simulink model "TQ2m"  (Simulink 8.0)
settings: Solver=FixedStepDiscrete  StartTime=0.0  StopTime=inf  FixedStep=0.0025  RelTol=1e-3
undefined symbols (not defined in the file): Serial_Port, Standard_Devices
libraries: simulink x2, rtwinlib x2
Description:
  | Vectorized Quantizer C-MEX S-function
settings Model: Creator=The MathWorks Inc.  LastModifiedBy=x  SimulationMode=external  ExtModeTrigDuration=10000
settings SolverCC: PositivePriorityOrder=on
settings DataIOCC: LimitDataPoints=off  SignalLoggingSaveFormat=ModelDataLogs
settings OptimizationCC: BlockReduction=off  BooleanDataType=off  InitFltsAndDblsToZero=on
settings DebuggingCC: SaveWithParameterizedLinksMsg=none  SignalResolutionControl=TryResolveAllWithWarning  SolverPrmCheckMsg=none  MultiTaskDSMMsg=warning  MultiTaskCondExecSysMsg=none  FcnCallInpInsideContextMsg=UseLocalSettings
settings HardwareCC: ProdIntDivRoundTo=Zero  ProdEndianess=LittleEndian  ProdHWDeviceType=Generic->32-bit x86 compatible  TargetIntDivRoundTo=Zero  TargetEndianess=LittleEndian  TargetHWDeviceType=MATLAB Host  ProdEqTarget=off
settings SFSimCC: SimCustomHeaderCode=|
  | advapi32.dll
  | comctl32.dll
  | comdlg32.dll
  | gdi32.dll
  | kernel32.dll
  | netapi32.dll
  | shell32.dll
  | shlwapi.dll
  | user32.dll
  | WindowsCodecs.dll
settings SFSimCC: SimUserLibraries=|
  | NtDsAPI.Lib
  | NTMSAPI.Lib
  | NtQuery.Lib
  | windowscodecs.lib
settings RTWCC: SystemTargetFile=rtwin.tlc  TemplateMakefile=rtwin.tmf  Description=Real-Time Windows Target  ProcessScript=rtwin_make_rtw_hook  IncludeERTFirstTime=on  RTWCompilerOptimization=On
settings RTWCC: CustomLibrary=|
  | kernel32.lib
  | kernel32.dll
settings CodeAppCC: MaxIdLength=95  CustomSymbolStrType=$N$R$M_T  InternalIdentifier=Shortened
settings RTWinTargetCC: TargetLibSuffix=_rtwin.lib  TargetPreCompLibLocation=C:\Program Files\MATLAB\R2012b\toolbox\rtw\targets\rtwin\lib\win64  CodeReplacementLibrary=ANSI_C  RTWinDir=C:/PROGRA~1/MATLAB/R2012b/toolbox/rtw/targets/rtwin  TargetArch=win64

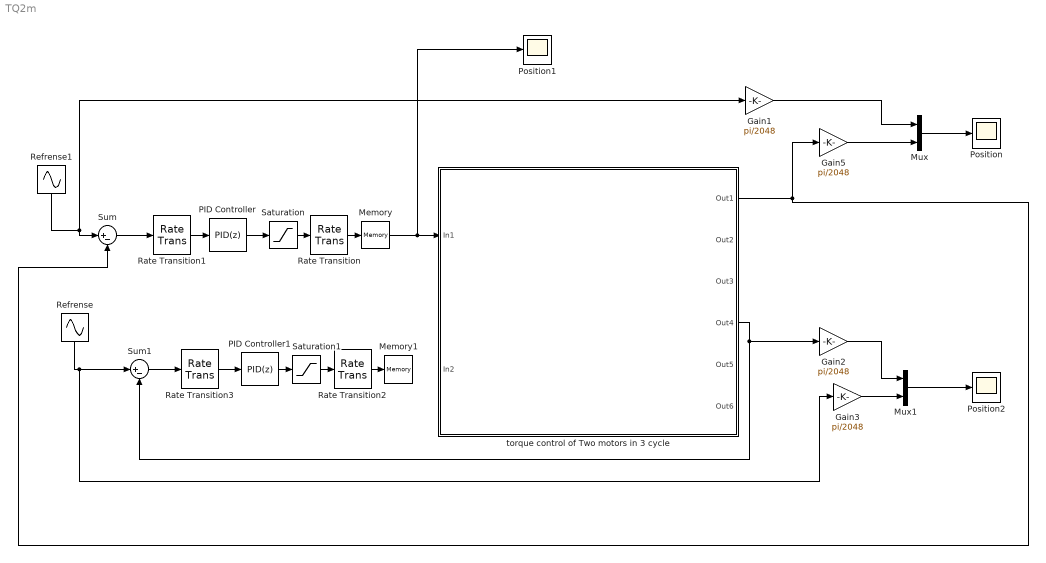
== system TQ2m ==
  Gain{1..3,5} (4 alike) : Gain  Gain=pi/2048
  Memory : Memory
  Memory1 : Memory
  Mux : Mux  Inputs=2
  Mux1 : Mux  Inputs=2
  PID Controller : simulink/Continuous/PID Controller  Controller=PID  TimeDomain=Discrete-time  SampleTime=0.01  IntegratorMethod=Forward Euler  FilterMethod=Forward Euler  Form=Parallel  P=0.002  I=0.01  D=0.00005  N=100  InitialConditionSource=internal  InitialConditionForIntegrator=0  InitialConditionForFilter=0  ExternalReset=none  LimitOutput=off  UpperSaturationLimit=inf  LowerSaturationLimit=-inf  LinearizeAsGain=on  AntiWindupMode=none  Kb=1  TrackingMode=off  Kt=1  PParamMin=[]  PParamMax=[]  IParamMin=[]  IParamMax=[]  DParamMin=[]  DParamMax=[]  NParamMin=[]  NParamMax=[]  KbParamMin=[]  KbParamMax=[]  KtParamMin=[]  KtParamMax=[]  POutMin=[]  POutMax=[]  IOutMin=[]  IOutMax=[]  DOutMin=[]  DOutMax=[]  NOutMin=[]  NOutMax=[]  KbOutMin=[]  KbOutMax=[]  KtOutMin=[]  KtOutMax=[]  IntegratorOutMin=[]  IntegratorOutMax=[]  FilterOutMin=[]  FilterOutMax=[]  SumOutMin=[]  SumOutMax=[]  SumI1OutMin=[]  SumI1OutMax=[]  SumI2OutMin=[]  SumI2OutMax=[]  SumI3OutMin=[]  SumI3OutMax=[]  SumDOutMin=[]  SumDOutMax=[]  SaturationOutMin=[]  SaturationOutMax=[]  IntegratorContinuousStateAttributes=''  IntegratorStateMustResolveToSignalObject=off  IntegratorRTWStateStorageClass=Auto  FilterContinuousStateAttributes=''  FilterStateMustResolveToSignalObject=off  FilterRTWStateStorageClass=Auto
      link override Filter: IntegratorMethod=Integration: Forward Euler  gainval=1.0  ExternalReset=none  InitialConditionSource=internal  InitialCondition=InitialConditionForFilter  InitialConditionMode=State only (most efficient)  SampleTime=-1  OutMin=FilterOutMin  OutMax=FilterOutMax  OutDataTypeStr=FilterOutDataTypeStr  LimitOutput=off  UpperSaturationLimit=inf  LowerSaturationLimit=-inf  ShowSaturationPort=off  ShowStatePort=off
      link override Filter: StateMustResolveToSignalObject=off  RTWStateStorageClass=Auto
  PID Controller1 : simulink/Continuous/PID Controller  Controller=PID  TimeDomain=Discrete-time  SampleTime=0.01  IntegratorMethod=Forward Euler  FilterMethod=Forward Euler  Form=Parallel  P=0.002  I=0.01  D=0.00005  N=100  InitialConditionSource=internal  InitialConditionForIntegrator=0  InitialConditionForFilter=0  ExternalReset=none  LimitOutput=off  UpperSaturationLimit=inf  LowerSaturationLimit=-inf  LinearizeAsGain=on  AntiWindupMode=none  Kb=1  TrackingMode=off  Kt=1  PParamMin=[]  PParamMax=[]  IParamMin=[]  IParamMax=[]  DParamMin=[]  DParamMax=[]  NParamMin=[]  NParamMax=[]  KbParamMin=[]  KbParamMax=[]  KtParamMin=[]  KtParamMax=[]  POutMin=[]  POutMax=[]  IOutMin=[]  IOutMax=[]  DOutMin=[]  DOutMax=[]  NOutMin=[]  NOutMax=[]  KbOutMin=[]  KbOutMax=[]  KtOutMin=[]  KtOutMax=[]  IntegratorOutMin=[]  IntegratorOutMax=[]  FilterOutMin=[]  FilterOutMax=[]  SumOutMin=[]  SumOutMax=[]  SumI1OutMin=[]  SumI1OutMax=[]  SumI2OutMin=[]  SumI2OutMax=[]  SumI3OutMin=[]  SumI3OutMax=[]  SumDOutMin=[]  SumDOutMax=[]  SaturationOutMin=[]  SaturationOutMax=[]  IntegratorContinuousStateAttributes=''  IntegratorStateMustResolveToSignalObject=off  IntegratorRTWStateStorageClass=Auto  FilterContinuousStateAttributes=''  FilterStateMustResolveToSignalObject=off  FilterRTWStateStorageClass=Auto
      link override Filter: IntegratorMethod=Integration: Forward Euler  gainval=1.0  ExternalReset=none  InitialConditionSource=internal  InitialCondition=InitialConditionForFilter  InitialConditionMode=State only (most efficient)  SampleTime=-1  OutMin=FilterOutMin  OutMax=FilterOutMax  OutDataTypeStr=FilterOutDataTypeStr  LimitOutput=off  UpperSaturationLimit=inf  LowerSaturationLimit=-inf  ShowSaturationPort=off  ShowStatePort=off
      link override Filter: StateMustResolveToSignalObject=off  RTWStateStorageClass=Auto
  Position : Scope
      settings: TimeRange=10  YMin=2.2  YMax=3.9  SaveName=ScopeData5
  Position1 : Scope
      settings: TimeRange=10  YMin=-0.3  YMax=0.25
  Position2 : Scope
      settings: TimeRange=10  YMin=2.3  YMax=3.9  SaveName=ScopeData9
  Rate Transition : RateTransition
  Rate Transition1 : RateTransition  OutPortSampleTime=0.01
  Rate Transition2 : RateTransition
  Rate Transition3 : RateTransition  OutPortSampleTime=0.01
  Refrense : Sin  Amplitude=500  Bias=2000  Frequency=1.5
  Refrense1 : Sin  Amplitude=500  Bias=2000  Frequency=1.5
  Saturation : Saturate  UpperLimit=6  LowerLimit=-6
  Saturation1 : Saturate  UpperLimit=6  LowerLimit=-6
  Sum : Sum  Inputs=|+-
  Sum1 : Sum  Inputs=|+-
  torque control of Two motors in 3 cycle : Subsystem  TreatAsAtomicUnit=on  mask(MX64R Real Time Windows Target){p1=3, p2=1}
      mask prompts: p1 "Dynamixel ID 1"; p2 "Dynamixel ID 2"
      mask help:
      | This Block is desined for torque control of two Dynamixel motor (MX64R )in real time workshop
      | please be advised with the following issue:
      | Caution1>> change Status Return Level to 1 in EEprom inorder to receive status packet just for read command.
      | Caution2>> It is recommended that Return Delay Time be set as the minimum value within the allowed range of Main Controller.
      | Caution3>> Total sample time for 2 motors is equal to Ts/3. (Ts is the simulink sample time)
      | Copyright @ Aras Lab.
      mask Display:
      | image(imread('mx64RR.jpg'))
      | port_label('input',1,'Torque1')
      | port_label('input',2,'Torque2')
      | port_label('output',1,'position1')
      | port_label('output',2,'velovity1')
      | port_label('output',3,'load1')
      | port_label('output',4,'position2')
      | port_label('output',5,'velovity2')
      | port_label('output',6,'load2')
  wires:
  Sum/1 -> Rate Transition1/1
  PID Controller/1 -> Saturation/1
  Saturation/1 -> Rate Transition/1
  Rate Transition/1 -> Memory/1
  Rate Transition1/1 -> PID Controller/1
  Mux/1 -> Position/1
  Refrense1/1 -> Sum/1, Gain1/1
  torque control of Two motors in 3 cycle/1(Out1) -> Sum/2, Gain5/1
  Gain1/1 -> Mux/1
  Sum1/1 -> Rate Transition3/1
  PID Controller1/1 -> Saturation1/1
  Saturation1/1 -> Rate Transition2/1
  Rate Transition2/1 -> Memory1/1
  Rate Transition3/1 -> PID Controller1/1
  Refrense/1 -> Gain3/1, Sum1/1
  Mux1/1 -> Position2/1
  torque control of Two motors in 3 cycle/4(Out4) -> Sum1/2, Gain2/1
  Gain3/1 -> Mux1/2
  Gain5/1 -> Mux/2
  Gain2/1 -> Mux1/1
  Memory/1 -> Position1/1, torque control of Two motors in 3 cycle/1(In1)

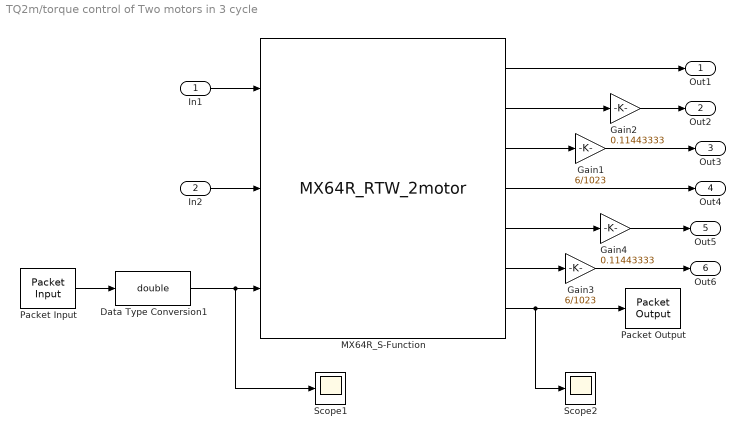
== system TQ2m/torque control of Two motors in 3 cycle ==
  In1 : Inport
  In2 : Inport  Port=2
  Data Type Conversion1 : DataTypeConversion  OutDataTypeStr=double  ConvertRealWorld=Stored Integer (SI)
  Gain1 : Gain  Gain=6/1023
  Gain2 : Gain  Gain=0.11443333
  Gain3 : Gain  Gain=6/1023
  Gain4 : Gain  Gain=0.11443333
  MX64R_S-Function : S-Function  FunctionName=MX64R_RTW_2motor  Parameters=p1,p2  EnableBusSupport=off  mask(S-function: MX64R_RTW2){}
      mask Display:
      | port_label('input',1,'desire torque1')
      | port_label('input',2,'desire torque2')
      | port_label('input',3,'serial in')
      | port_label('output',1,'position1')
      | port_label('output',2,'velocity1')
      | port_label('output',3,'load1')
      | port_label('output',4,'position2')
      | port_label('output',5,'velocity2')
      | port_label('output',6,'load2')
      | port_label('output',7,'serial out')
  Packet Input : rtwinlib/Packet Input  SampleTime=-1  MaxMissedTicks=25  ShowMissedTicks=off  YieldWhenWaiting=off  DrvName=Standard_Devices/Serial_Port  DrvAddress=3  DrvOptions=[3000000 8 0 0 0 1 0 0]  PacketSize=12  DataTypes='12*uint8'  ShowReady=off  ShowError=off  PacketID=1  ByteOrder=1  ShowTimestamp=off
      settings: AttributesFormatString=Standard Devices\nSerial Port [3h]
  Packet Output : rtwinlib/Packet Output  SampleTime=-1  MaxMissedTicks=25  ShowMissedTicks=off  YieldWhenWaiting=off  DrvName=Standard_Devices/Serial_Port  DrvAddress=3  DrvOptions=[3000000 8 0 0 0 1 0 0]  PacketSize=16  DataTypes='16*uint8'  ShowReady=off  ShowError=off  PacketID=1  ByteOrder=1  InitialValue=[]  FinalValue=[]
      settings: AttributesFormatString=Standard Devices\nSerial Port [3h]
  Scope1 : Scope
      settings: TimeRange=10  YMin=0  YMax=275  SaveName=ScopeData2
  Scope2 : Scope
      settings: TimeRange=10  YMin=0  YMax=275  SaveName=ScopeData3
  Out1 : Outport  OutMin=[0]  OutMax=[2*pi]
  Out2 : Outport  Port=2
  Out3 : Outport  Port=3
  Out4 : Outport  Port=4  OutMin=[0]  OutMax=[2*pi]
  Out5 : Outport  Port=5
  Out6 : Outport  Port=6
  wires:
  In1/1 -> MX64R_S-Function/1
  Packet Input/1 -> Data Type Conversion1/1
  Data Type Conversion1/1 -> MX64R_S-Function/3, Scope1/1
  MX64R_S-Function/2 -> Gain2/1
  MX64R_S-Function/3 -> Gain1/1
  MX64R_S-Function/1 -> Out1/1
  Gain1/1 -> Out3/1
  Gain2/1 -> Out2/1
  MX64R_S-Function/5 -> Gain4/1
  MX64R_S-Function/6 -> Gain3/1
  MX64R_S-Function/4 -> Out4/1
  Gain3/1 -> Out6/1
  Gain4/1 -> Out5/1
  MX64R_S-Function/7 -> Scope2/1, Packet Output/1
  In2/1 -> MX64R_S-Function/2
